simulink model "modelOnRealCar"  (R2015b)
settings: Solver=FixedStepDiscrete  StartTime=0.0  StopTime=inf  RelTol=1e-3
values from neighbouring files (symbols this model uses):
  differenziale = 0.01*vel_mot    (= 0.005)    [parametri_modello.m]
  esposizione = 200    [parametri_modello.m]
  rallenta = 1/20    (= 0.05)    [parametri_modello.m]
  vel_mot = 0.5    [parametri_modello.m]
undefined symbols (not defined in the file or in its folder): DiscIntNeverNeededParam
libraries: frdmtfcshieldlib x11, simulink x2
settings Model: Creator=The MathWorks Inc.  LastModifiedBy=dgc14
settings DataIOCC: SaveFormat=Array
settings OptimizationCC: OptimizeModelRefInitCode=on  LifeSpan=1  MaxStackSize=64
settings DebuggingCC: SolverPrmCheckMsg=warning  ParameterPrecisionLossMsg=none
settings HardwareCC: ProdBitPerPointer=32  ProdLargestAtomicInteger=Long  ProdLargestAtomicFloat=Double  ProdIntDivRoundTo=Undefined  ProdWordSize=32  ProdHWDeviceType=ARM Compatible->ARM Cortex
settings RTWCC: SystemTargetFile=ert.tlc  TemplateMakefile=ert_default_tmf  Description=Embedded Coder  Toolchain=GNU Tools for ARM Embedded Processors
settings CodeAppCC: IgnoreCustomStorageClasses=off
settings ConfigComp: CovModelRefEnable=Off  CovSFcnEnable=off

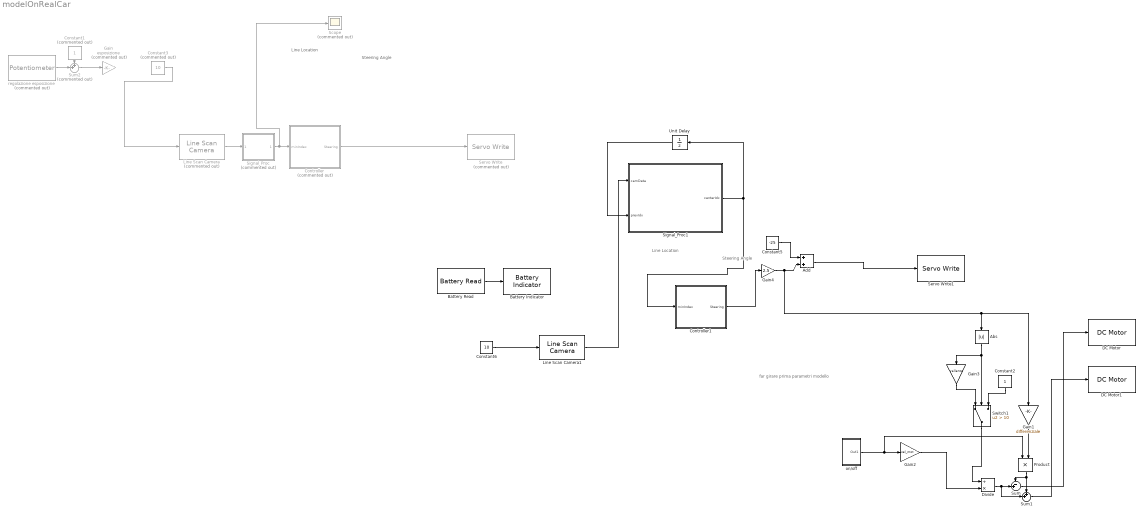
== system modelOnRealCar ==
  note: far girare prima parametri modello
  note: Steering
      | Angle
  note: Line Location
  note: Steering
      | Angle
  note: Line Location
  Abs : Abs
  Add : Sum
  Battery Indicator : frdmtfcshieldlib/Battery Indicator
  Battery Read : frdmtfcshieldlib/Battery Read  SampleTime=0.1
  Constant1 : Constant  Commented=on
  Constant2 : Constant
  Constant3 : Constant  Commented=on  Value=10
  Constant5 : Constant  Value=-25
  Constant6 : Constant  Value=10
  Controller : Subsystem  Commented=on
  Controller1 : Subsystem
  DC Motor : frdmtfcshieldlib/DC Motor  WhichMotor=A
  DC Motor1 : frdmtfcshieldlib/DC Motor  WhichMotor=B
  Divide : Product  Inputs=/*
  Gain : Gain  Commented=on  Gain=esposizione
  Gain1 : Gain  Gain=differenziale
  Gain2 : Gain  Gain=vel_mot
  Gain3 : Gain  Gain=rallenta
  Gain4 : Gain  Gain=2.5
  Line Scan Camera : frdmtfcshieldlib/Line Scan Camera  Commented=on  CameraHeader=0  SampleTime=0.01
  Line Scan Camera1 : frdmtfcshieldlib/Line Scan Camera  CameraHeader=0  SampleTime=0.01
  Product : Product
  Scope : Scope  Commented=on
  Servo Write : frdmtfcshieldlib/Servo Write  Commented=on  WhichServo=0  minAngle=-40  maxAngle=40
  Servo Write1 : frdmtfcshieldlib/Servo Write  WhichServo=0  minAngle=-40  maxAngle=40
  Signal_Proc : MATLAB Function  Commented=on  TreatAsAtomicUnit=on
  Signal_Proc1 : MATLAB Function  TreatAsAtomicUnit=on
  Sum : Sum  Inputs=-+|
  Sum1 : Sum  Inputs=++|
  Sum2 : Sum  Commented=on  Inputs=++|
  Switch1 : Switch  Criteria=u2 > Threshold  Threshold=10
  Unit Delay : UnitDelay  SampleTime=-1
  "on/off " : Subsystem
  regolazione esposizione : frdmtfcshieldlib/Potentiometer  Commented=on  WhichPot=A  SampleTime=0.01
  wires:
  Line Scan Camera/1 -> Signal_Proc/1(camData)
  Battery Read/1 -> Battery Indicator/1
  Controller/1(Steering) -> Servo Write/1
  Product/1 -> Sum/1, Sum1/1
  Divide/1 -> Sum1/2, Sum/2
  Gain1/1 -> Product/2
  Abs/1 -> Gain3/1, Switch1/2
  Constant2/1 -> Switch1/3
  Gain3/1 -> Switch1/1
  Switch1/1 -> Divide/1
  Gain2/1 -> Divide/2
  "on/off "/1(Out1) -> Product/1, Gain2/1
  Constant1/1 -> Sum2/1
  regolazione esposizione/1 -> Sum2/2
  Sum2/1 -> Gain/1
  Constant3/1 -> Line Scan Camera/1
  Signal_Proc/1(centerIdx) -> Scope/1, Controller/1(minIndex)
  Line Scan Camera1/1 -> Signal_Proc1/1(camData)
  Constant6/1 -> Line Scan Camera1/1
  Signal_Proc1/1(centerIdx) -> Unit Delay/1, Controller1/1(minIndex)
  Constant5/1 -> Add/1
  Controller1/1(Steering) -> Gain4/1
  Gain4/1 -> Gain1/1, Abs/1, Add/2
  Add/1 -> Servo Write1/1
  Unit Delay/1 -> Signal_Proc1/2(prevIdx)
  Sum/1 -> DC Motor/1
  Sum1/1 -> DC Motor1/1

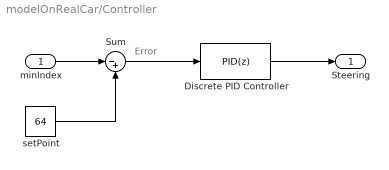
== system modelOnRealCar/Controller ==
  note: Error
  minIndex : Inport
  Discrete PID Controller : simulink/Continuous/PID Controller  Controller=PID  TimeDomain=Discrete-time  SampleTime=-1  IntegratorMethod=Trapezoidal  FilterMethod=Forward Euler  Form=Ideal  UseFilter=on  ControllerParametersSource=internal  P=0.32  I=0.001  D=0.01  N=100  InitialConditionSource=internal  InitialConditionForIntegrator=0  InitialConditionForFilter=0  ExternalReset=none  LimitOutput=on  UpperSaturationLimit=37  LowerSaturationLimit=-37  LinearizeAsGain=off  AntiWindupMode=none  Kb=1  TrackingMode=off  Kt=1  PParamMin=[]  PParamMax=[]  IParamMin=[]  IParamMax=[]  DParamMin=[]  DParamMax=[]  NParamMin=[]  NParamMax=[]  KbParamMin=[]  KbParamMax=[]  KtParamMin=[]  KtParamMax=[]  POutMin=[]  POutMax=[]  IOutMin=[]  IOutMax=[]  DOutMin=[]  DOutMax=[]  NOutMin=[]  NOutMax=[]  KbOutMin=[]  KbOutMax=[]  KtOutMin=[]  KtOutMax=[]  IntegratorOutMin=[]  IntegratorOutMax=[]  FilterOutMin=[]  FilterOutMax=[]  SumOutMin=[]  SumOutMax=[]  SumI1OutMin=[]  SumI1OutMax=[]  SumI2OutMin=[]  SumI2OutMax=[]  SumI3OutMin=[]  SumI3OutMax=[]  SumDOutMin=[]  SumDOutMax=[]  SaturationOutMin=[]  SaturationOutMax=[]  IntegratorContinuousStateAttributes=''  IntegratorStateMustResolveToSignalObject=off  IntegratorRTWStateStorageClass=Auto  FilterContinuousStateAttributes=''  FilterStateMustResolveToSignalObject=off  FilterRTWStateStorageClass=Auto  DifferentiatorICPrevScaledInput=0  DifferentiatorOutMin=[]  DifferentiatorOutMax=[]
  Sum : Sum  Inputs=|-+
  setPoint : Constant  Value=64
  Steering : Outport
  wires:
  setPoint/1 -> Sum/2
  minIndex/1 -> Sum/1
  Discrete PID Controller/1 -> Steering/1
  Sum/1 -> Discrete PID Controller/1

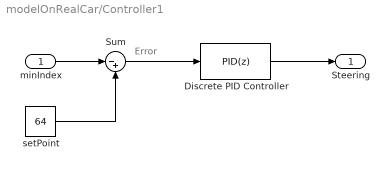
== system modelOnRealCar/Controller1 ==
  note: Error
  minIndex : Inport
  Discrete PID Controller : simulink/Continuous/PID Controller  Controller=PID  TimeDomain=Discrete-time  SampleTime=-1  IntegratorMethod=Trapezoidal  FilterMethod=Forward Euler  Form=Ideal  UseFilter=on  ControllerParametersSource=internal  P=0.32  I=0.001  D=0.01  N=100  InitialConditionSource=internal  InitialConditionForIntegrator=0  InitialConditionForFilter=0  ExternalReset=none  LimitOutput=on  UpperSaturationLimit=37  LowerSaturationLimit=-37  LinearizeAsGain=off  AntiWindupMode=none  Kb=1  TrackingMode=off  Kt=1  PParamMin=[]  PParamMax=[]  IParamMin=[]  IParamMax=[]  DParamMin=[]  DParamMax=[]  NParamMin=[]  NParamMax=[]  KbParamMin=[]  KbParamMax=[]  KtParamMin=[]  KtParamMax=[]  POutMin=[]  POutMax=[]  IOutMin=[]  IOutMax=[]  DOutMin=[]  DOutMax=[]  NOutMin=[]  NOutMax=[]  KbOutMin=[]  KbOutMax=[]  KtOutMin=[]  KtOutMax=[]  IntegratorOutMin=[]  IntegratorOutMax=[]  FilterOutMin=[]  FilterOutMax=[]  SumOutMin=[]  SumOutMax=[]  SumI1OutMin=[]  SumI1OutMax=[]  SumI2OutMin=[]  SumI2OutMax=[]  SumI3OutMin=[]  SumI3OutMax=[]  SumDOutMin=[]  SumDOutMax=[]  SaturationOutMin=[]  SaturationOutMax=[]  IntegratorContinuousStateAttributes=''  IntegratorStateMustResolveToSignalObject=off  IntegratorRTWStateStorageClass=Auto  FilterContinuousStateAttributes=''  FilterStateMustResolveToSignalObject=off  FilterRTWStateStorageClass=Auto  DifferentiatorICPrevScaledInput=0  DifferentiatorOutMin=[]  DifferentiatorOutMax=[]
  Sum : Sum  Inputs=|-+
  setPoint : Constant  Value=64
  Steering : Outport
  wires:
  setPoint/1 -> Sum/2
  minIndex/1 -> Sum/1
  Discrete PID Controller/1 -> Steering/1
  Sum/1 -> Discrete PID Controller/1

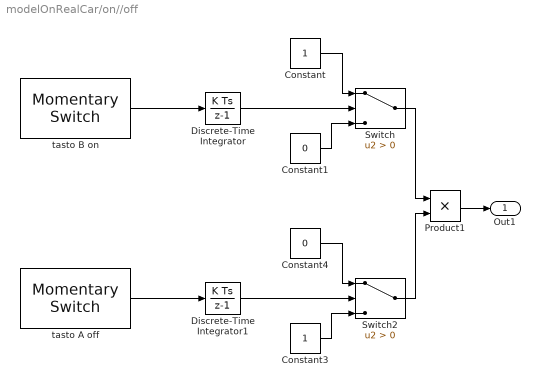
== system modelOnRealCar/on//off  ==
  Constant : Constant
  Constant1 : Constant  Value=0
  Constant3 : Constant
  Constant4 : Constant  Value=0
  Discrete-Time Integrator : DiscreteIntegrator  SampleTime=0.01  ICPrevOutput=DiscIntNeverNeededParam  ICPrevScaledInput=DiscIntNeverNeededParam
  Discrete-Time Integrator1 : DiscreteIntegrator  SampleTime=0.01  ICPrevOutput=DiscIntNeverNeededParam  ICPrevScaledInput=DiscIntNeverNeededParam
  Product1 : Product
  Switch : Switch  Criteria=u2 > Threshold
  Switch2 : Switch  Criteria=u2 > Threshold
  tasto A off : frdmtfcshieldlib/Momentary Switch  WhichSwitch=A  SampleTime=0.01
  tasto B on : frdmtfcshieldlib/Momentary Switch  WhichSwitch=B  SampleTime=0.01
  Out1 : Outport
  wires:
  Switch2/1 -> Product1/2
  Product1/1 -> Out1/1
  Constant1/1 -> Switch/3
  Constant/1 -> Switch/1
  tasto B on/1 -> Discrete-Time Integrator/1
  Switch/1 -> Product1/1
  Discrete-Time Integrator/1 -> Switch/2
  Discrete-Time Integrator1/1 -> Switch2/2
  Constant4/1 -> Switch2/1
  Constant3/1 -> Switch2/3
  tasto A off/1 -> Discrete-Time Integrator1/1

== matlab function modelOnRealCar/Signal_Proc1 ==
  data: centerIdx output; camData input; prevIdx input
function centerIdx  = centerTrackIdx(camData, prevIdx)

camData = camData(1:118);
threshold = (max(camData)+min(camData))/2;
black = zeros(length(camData),1);
j = 1;
for i=1:length(camData)
    if(camData(i)<threshold)
        black(j)=i;
        j = j+1;
    end
end
j = j-1;
if(j~=0)
    centerIdx = black(floor(j/2));
else
    centerIdx = prevIdx;
end

%%%%%%%%%%%%%%%%%%%%%%%%%%%%%%%%%%%%%%%%%%%%%%%%%%%%%%%%%%%%%%%%%%%%%%%%%%%%%%%%%%%

%find STOP
% 
% h = 29;%camera high
% a = 29.21;%cm (3'-1/2") length from lateral line to center track
% b=60;
% camera_error = 7;
% d = sqrt(b^2+h^2);%diagonal length from camera to view center point
% alfa = atan2(a,d);%optical angle from center to lateral line
% pixel_gap = round(alfa/0.007604262);%pixel from lateral line to center track
% pixel_edge = 64 - pixel_gap + camera_error;%pixel from lateral line to outdoor track
% s1 = 3.81;%cm [1 1/2"] center track to begin stop
% s2 = 13.97;%cm [5 1/2"] center track to end stop
% alfa1 = atan2(s1,d);
% alfa2 = atan2(s2,d);
% s1_pixel = round(alfa1/0.007604262);
% s2_pixel = round(alfa2/0.007604262);
% 
% 
% 
% %         if length(find(camData(64-s2_pixel:64-s1_pixel) < threshold)) > 0.1*(s2_pixel-s1_pixel) &&...
% %             length(find(camData(64+s1_pixel:64+s2_pixel) < threshold)) > 0.1*(s2_pixel-s1_pixel) &&...
% %             length(find(camData(64-s1_pixel:64+s1_pixel) > threshold)) > 0.1*2*s1_pixel
% 
% if length(find(camData(64-s2_pixel-10:64-s1_pixel+10) < threshold)) > 0.6*(s2_pixel-s1_pixel) &&...
%     length(find(camData(64+s1_pixel-10:64+s2_pixel+10) < threshold)) > 0.6*(s2_pixel-s1_pixel) &&...
%     length(find(camData(64-s1_pixel-10:64+s1_pixel+10) > threshold)) > 2*s1_pixel
% 
% %         if length(find(camData(30:98) < threshold)) > (s2_pixel-s1_pixel) &&...
% %             length(find(camData(64-s1_pixel:64+s1_pixel) > threshold)) > 0.1*2*s1_pixel
% 
%     stop = 1;
%     centerIdx=64;
% end
% 
% if length(find(camData(40:60) < threshold)) > 0.55*20 &&...
%     length(find(camData(70:90) < threshold)) > 0.55*20 &&...
%     length(find(camData(60:70) > threshold)) > 0.55*10
% 
% %         if length(find(camData(30:98) < threshold)) > (s2_pixel-s1_pixel) &&...
% %             length(find(camData(64-s1_pixel:64+s1_pixel) > threshold)) > 0.1*2*s1_pixel
% 
%     stop = 1;
%     centerIdx=64;
% end

== matlab function modelOnRealCar/Signal_Proc ==
  data: centerIdx output; camData input
function centerIdx  = centerTrackIdx(camData)

threshold = 5e4;
black = zeros(length(camData),1);
j = 1;
for i=1:length(camData)
    if(camData(i)<threshold)
        black(j)=i;
        j = j+1;
    end
end
j = j-1;
if(j~=0)
    centerIdx = black(floor(j/2));
else
    centerIdx = 64;
end

%%%%%%%%%%%%%%%%%%%%%%%%%%%%%%%%%%%%%%%%%%%%%%%%%%%%%%%%%%%%%%%%%%%%%%%%%%%%%%%%%%%

%find STOP
% 
% h = 29;%camera high
% a = 29.21;%cm (3'-1/2") length from lateral line to center track
% b=60;
% camera_error = 7;
% d = sqrt(b^2+h^2);%diagonal length from camera to view center point
% alfa = atan2(a,d);%optical angle from center to lateral line
% pixel_gap = round(alfa/0.007604262);%pixel from lateral line to center track
% pixel_edge = 64 - pixel_gap + camera_error;%pixel from lateral line to outdoor track
% s1 = 3.81;%cm [1 1/2"] center track to begin stop
% s2 = 13.97;%cm [5 1/2"] center track to end stop
% alfa1 = atan2(s1,d);
% alfa2 = atan2(s2,d);
% s1_pixel = round(alfa1/0.007604262);
% s2_pixel = round(alfa2/0.007604262);
% 
% 
% 
% %         if length(find(camData(64-s2_pixel:64-s1_pixel) < threshold)) > 0.1*(s2_pixel-s1_pixel) &&...
% %             length(find(camData(64+s1_pixel:64+s2_pixel) < threshold)) > 0.1*(s2_pixel-s1_pixel) &&...
% %             length(find(camData(64-s1_pixel:64+s1_pixel) > threshold)) > 0.1*2*s1_pixel
% 
% if length(find(camData(64-s2_pixel-10:64-s1_pixel+10) < threshold)) > 0.6*(s2_pixel-s1_pixel) &&...
%     length(find(camData(64+s1_pixel-10:64+s2_pixel+10) < threshold)) > 0.6*(s2_pixel-s1_pixel) &&...
%     length(find(camData(64-s1_pixel-10:64+s1_pixel+10) > threshold)) > 2*s1_pixel
% 
% %         if length(find(camData(30:98) < threshold)) > (s2_pixel-s1_pixel) &&...
% %             length(find(camData(64-s1_pixel:64+s1_pixel) > threshold)) > 0.1*2*s1_pixel
% 
%     stop = 1;
%     centerIdx=64;
% end
% 
% if length(find(camData(40:60) < threshold)) > 0.55*20 &&...
%     length(find(camData(70:90) < threshold)) > 0.55*20 &&...
%     length(find(camData(60:70) > threshold)) > 0.55*10
% 
% %         if length(find(camData(30:98) < threshold)) > (s2_pixel-s1_pixel) &&...
% %             length(find(camData(64-s1_pixel:64+s1_pixel) > threshold)) > 0.1*2*s1_pixel
% 
%     stop = 1;
%     centerIdx=64;
% end
